simulink model "P3_Ex12"  (R2021a)
settings: Solver=FixedStepAuto  StartTime=0.0  StopTime=Total_time  RelTol=1e-3
PreLoadFcn:
  | Preload11_12
values from neighbouring files (symbols this model uses):
  Kd = x(4)*Ts    [P3_Ex11code.m]    (also in Preload11_12.m = 0)
  Ki = x(3)*2/Ts    [P3_Ex11code.m]    (also in Preload11_12.m = 0)
  Kp = x(2)    [P3_Ex11code.m]    (also in Preload11_12.m = 1)
  Ts = 0.01    [P3_Ex11code.m]    (also in Preload11_12.m)
undefined symbols (not defined in the file or in its folder): DiscIntNeverNeededParam
libraries: arduinolib x4, simulink x3
settings Model: SimulationMode=external  ExtModeTrigDuration=2  Creator=Eneko Lerma  LastModifiedBy=UPCnet
settings SolverCC: AlgebraicLoopSolver=TrustRegion
settings DataIOCC: ReturnWorkspaceOutputs=off
settings OptimizationCC: EnhancedBackFolding=on  PassReuseOutputArgsAs=Individual arguments  MaxStackSize=64  OptimizeBlockOrder=speed  DifferentSizesBufferReuse=on  OptimizationCustomize=off  EfficientTunableParamExpr=on
settings DebuggingCC: ParameterPrecisionLossMsg=none  ParameterTunabilityLossMsg=error  SFMachineParentedDataDiag=warning  ArithmeticOperatorsInVariantConditions=warning
settings HardwareCC: ProdBitPerPointer=32  ProdBitPerSizeT=32  ProdBitPerPtrDiffT=32  ProdLargestAtomicInteger=Long  ProdLargestAtomicFloat=Double  ProdWordSize=32  ProdHWDeviceType=ARM Compatible->ARM Cortex
settings SFSimCC: SimUseLocalCustomCode=off  MATLABDynamicMemAlloc=off  CustomCodeUndefinedFunction=UseInterfaceOnly
settings RTWCC: SystemTargetFile=ert.tlc  HardwareBoard=Arduino Due  TemplateMakefile=ert_default_tmf  GenerateReport=on  RTWUseLocalCustomCode=off  Toolchain=Arduino ARM  BuildConfiguration=Faster Runs  IncludeHyperlinkInReport=on  LaunchReport=on  GenerateTraceInfo=on  GenerateTraceReport=on  GenerateTraceReportSl=on  GenerateTraceReportSf=on  GenerateTraceReportEml=on
settings RTWCC: CustomTerminator=|
  | writeDigitalPin((uint8_T)3, 0);
  | writeDigitalPin((uint8_T)5, 0);
settings CodeAppCC: ForceParamTrailComments=on  IgnoreCustomStorageClasses=off  OperatorAnnotations=on  SimulinkDataObjDesc=on  SFDataObjDesc=on  InsertBlockDesc=on
settings ERTTargetCC: SupportContinuousTime=on  SupportVariableSizeSignals=on

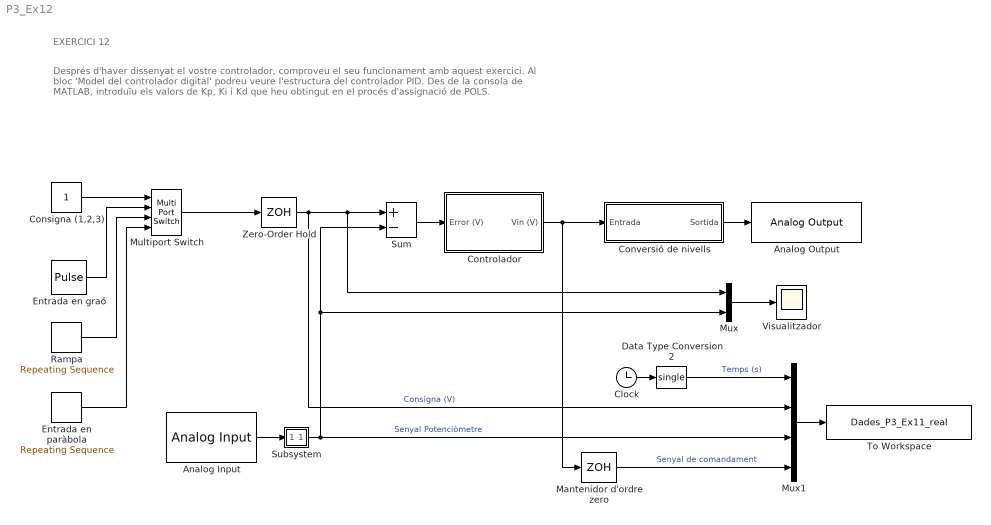
== system P3_Ex12 ==
  note: EXERCICI 12
  note: Després d'haver dissenyat el vostre controlador, comproveu el seu funcionament amb aquest exercici. Al bloc
      | 'Model del controlador digital' podreu veure l'estructura del controlador PID. Des de la consola de MATLAB, introduïu
      | els valors de Kp, Ki i Kd que heu obtingut en el procés d'assignació de POLS.
  Analog Input : arduinolib/Analog Input  pinNumber=1  ReadResultsOnly=off  ConversionTriggerSource=Software  ExternalTriggerType=uint32(0)  OutputDataType=uint16  EnableConversionCompleteNotify=off  EnableOuputStatus=off  SampleTime=0.005  blockPlatform=arduino
  Analog Output : arduinolib/Analog Output  DACpin=DAC1  blockPlatform=arduino
      settings: SourceProductBaseCode=ARDUINO
  Clock : Clock
  Consigna (1,2,3) : Constant
  Controlador : Subsystem
  Conversió de nivells : Subsystem
  Data Type Conversion2 : DataTypeConversion  OutDataTypeStr=single
  Entrada en paràbola : simulink/Sources/Repeating Sequence  rep_seq_t="[0    0.1000    0.2000    0.3000    0.4000    0.5000    0.6000    0.7000    0.8000 0.9000    1.0000    1.1000    1.2000    1.3000    1.4000    1.5000    1.6000    1.7000 1.8000    1.9000    2.0000    2.1000    2.2000    2.3000    2.4000    2.5000    2.6000 2.7000    2.8000    2.9000    3.0000    3.1000    3.2000    3.3000    3.4000    3.5000\t3.6000    3.7000    3.8000    3.9000    4.0000    4.1000    4.2000    4.3000    4.4000    4.5000    4.6000    4.7000    4.8000    4.9000    5.0000]"  rep_seq_y="[0    0.0008    0.0032    0.0072    0.0128    0.0200    0.0288    0.0392 0.0512    0.0648    0.0800    0.0968    0.1152    0.1352    0.1568    0.1800 0.2048    0.2312    0.2592    0.2888    0.3200    0.3528    0.3872    0.4232 0.4608    0.5000    0.5408    0.5832    0.6272    0.6728    0.7200    0.7688 0.8192    0.8712    0.9248    0.9800    1.0368    1.0952    1.1552    1.2168 1.2800    1.3448    1.4112    1.4792    1.5488    1.6200    1.6928    1.7672 1.8432    1.9208    2.0000]"
  Entrada en graó : DiscretePulseGenerator  PulseType=Time based  Amplitude=3.0  Period=18  PulseWidth=50  PhaseDelay=5
  Mantenidor d'ordre zero : ZeroOrderHold  SampleTime=Ts
  Multiport Switch : MultiPortSwitch  OutDataTypeStr=single
  Mux : Mux  Inputs=2
  Mux1 : Mux
  Rampa : simulink/Sources/Repeating Sequence  rep_seq_t="[0    0.1000    0.2000    0.3000    0.4000    0.5000    0.6000    0.7000    0.8000 0.9000    1.0000    1.1000    1.2000    1.3000    1.4000    1.5000    1.6000    1.7000 1.8000    1.9000    2.0000    2.1000    2.2000    2.3000    2.4000    2.5000    2.6000 2.7000    2.8000    2.9000    3.0000    3.1000    3.2000    3.3000    3.4000    3.5000\t3.6000    3.7000    3.8000    3.9000    4.0000    4.1000    4.2000    4.3000    4.4000    4.5000    4.6000    4.7000    4.8000    4.9000    5.0000]"  rep_seq_y=[-2.0000,-1.9200,-1.8400,-1.7600,-1.6800,-1.6000,-1.5200,-1.4400,-1.3600,-1.2800,-1.2000,-1.1200,-1.0400,-0.9600,-0.8800,-0.8000,-0.7200,-0.6400,-0.5600,-0.4800,-0.4000,-0.3200,-0.2400,-0.1600,-0.0800,0,0.0800,0.1600,0.2400,0.3200,0.4000,0.4800,0.5600,0.6400,0.7200,0.8000,0.8800,0.9600,1.0400,1.1200,1.2000,1.2800,1.3600,1.4400,1.5200,1.6000,1.6800,1.7600,1.8400,1.9200,2.0000]
  Subsystem : Subsystem
  Sum : Sum  Inputs=+-  AccumDataTypeStr=single
  To Workspace : ToWorkspace  VariableName=Dades_P3_Ex11_real  SampleTime=-1
  Visualitzador : Scope
  Zero-Order Hold : ZeroOrderHold  SampleTime=Ts
  wires:
  Mux/1 -> Visualitzador/1
  Sum/1 -> Controlador/1(Error (V))
  Conversió de nivells/1("  Sortida ") -> Analog Output/1
  Controlador/1(Vin (V)) -> Mantenidor d'ordre zero/1, Conversió de nivells/1(Entrada)
  Entrada en graó/1 -> Multiport Switch/2
  Consigna (1,2,3)/1 -> Multiport Switch/1
  Rampa/1 -> Multiport Switch/3
  Entrada en paràbola/1 -> Multiport Switch/4
  Zero-Order Hold/1 -> Sum/1, Mux/1, Mux1/2  "Consigna (V)"
  Mux1/1 -> To Workspace/1
  Mantenidor d'ordre zero/1 -> Mux1/4  "Senyal de comandament"
  Clock/1 -> Data Type Conversion2/1
  Multiport Switch/1 -> Zero-Order Hold/1
  Data Type Conversion2/1 -> Mux1/1  "Temps (s)"
  Subsystem/1("  ") -> Sum/2, Mux/2, Mux1/3  "Senyal Potenciòmetre"
  Analog Input/1 -> Subsystem/1(" ")

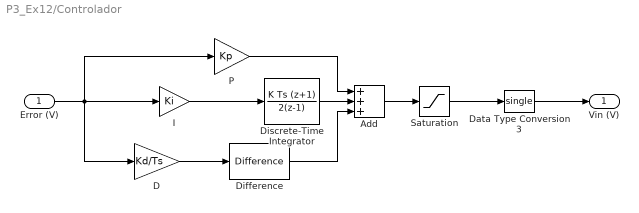
== system P3_Ex12/Controlador ==
  Error (V) : Inport
  Add : Sum  Inputs=+++  AccumDataTypeStr=single
  D : Gain  Gain=Kd/Ts
  Data Type Conversion3 : DataTypeConversion  OutDataTypeStr=single
  Difference : simulink/Discrete/Difference  ICPrevInput=0.0  OutMin=[]  OutMax=[]  OutDataType=fixdt(1, 16)  OutScaling=2^-10  DoSatur=off
  Discrete-Time Integrator : DiscreteIntegrator  IntegratorMethod=Integration: Trapezoidal  SampleTime=Ts  ICPrevOutput=DiscIntNeverNeededParam  ICPrevScaledInput=DiscIntNeverNeededParam
  I : Gain  Gain=Ki
  P : Gain  Gain=Kp
  Saturation : Saturate  UpperLimit=5  LowerLimit=-5  OutDataTypeStr=double
  Vin (V) : Outport  OutDataTypeStr=single  VectorParamsAs1DForOutWhenUnconnected=off
  wires:
  D/1 -> Difference/1
  P/1 -> Add/1
  Discrete-Time Integrator/1 -> Add/2
  I/1 -> Discrete-Time Integrator/1
  Add/1 -> Saturation/1
  Saturation/1 -> Data Type Conversion3/1
  Error (V)/1 -> I/1, P/1, D/1
  Data Type Conversion3/1 -> Vin (V)/1
  Difference/1 -> Add/3

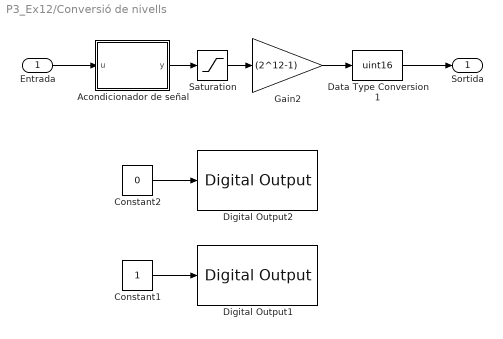
== system P3_Ex12/Conversió de nivells ==
  Entrada : Inport  OutDataTypeStr=single
  Acondicionador de señal : MATLAB Function  TreatAsAtomicUnit=on
  Constant1 : Constant
  Constant2 : Constant  Value=0
  Data Type Conversion1 : DataTypeConversion  OutDataTypeStr=uint16
  Digital Output1 : arduinolib/Digital Output  pinNumber=5  blockPlatform=arduino
  Digital Output2 : arduinolib/Digital Output  pinNumber=3  blockPlatform=arduino
  Gain2 : Gain  Gain=(2^12-1)  OutDataTypeStr=single
  Saturation : Saturate  UpperLimit=1  LowerLimit=0  OutDataTypeStr=single
  "  Sortida " : Outport  OutDataTypeStr=uint16  VectorParamsAs1DForOutWhenUnconnected=off
  wires:
  Gain2/1 -> Data Type Conversion1/1
  Entrada/1 -> Acondicionador de señal/1(u)
  Acondicionador de señal/1(y) -> Saturation/1
  Data Type Conversion1/1 -> "  Sortida "/1
  Saturation/1 -> Gain2/1
  Constant1/1 -> Digital Output1/1
  Constant2/1 -> Digital Output2/1

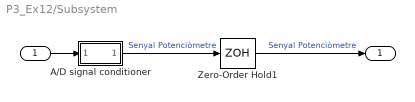
== system P3_Ex12/Subsystem ==
  " " : Inport
  A/D signal conditioner : Subsystem
  Zero-Order Hold1 : ZeroOrderHold  SampleTime=Ts
  "  " : Outport  VectorParamsAs1DForOutWhenUnconnected=off
  wires:
  A/D signal conditioner/1(" ") -> Zero-Order Hold1/1  "Senyal Potenciòmetre"
  Zero-Order Hold1/1 -> "  "/1  "Senyal Potenciòmetre"
  " "/1 -> A/D signal conditioner/1(" ")

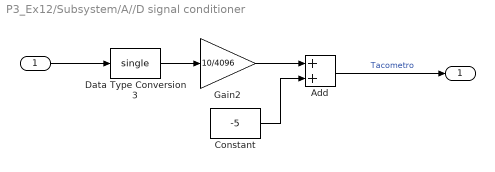
== system P3_Ex12/Subsystem/A//D signal conditioner ==
  " " : Inport
  Add : Sum  AccumDataTypeStr=single
  Constant : Constant  Value=-5  OutDataTypeStr=single
  Data Type Conversion3 : DataTypeConversion  OutDataTypeStr=single
  Gain2 : Gain  Gain=10/4096  OutDataTypeStr=single
  " " : Outport  VectorParamsAs1DForOutWhenUnconnected=off
  wires:
  Data Type Conversion3/1 -> Gain2/1
  Constant/1 -> Add/2
  Gain2/1 -> Add/1
  Add/1 -> " "/1  "Tacometro"
  " "/1 -> Data Type Conversion3/1

== matlab function P3_Ex12/Conversió de nivells/Acondicionador de señal ==
  data: u input; y output
function y = fcn(u)
y =0.0968*u+0.5058;
